simulink subsystem "complete_magnetic_model"  (R2023b)
settings: Solver=VariableStepAuto  StartTime=0.0  StopTime=10.0  RelTol=1e-3
undefined symbols (not defined in the file): astro_data, astroConstants, orbit_data, worldMag_data
settings Model: Creator=pierb  LastModifiedBy=pierb

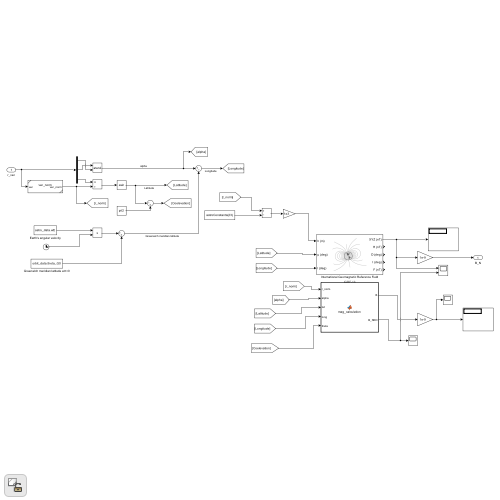
[thumbnail: Simulink's stored preview of the top-level diagram]
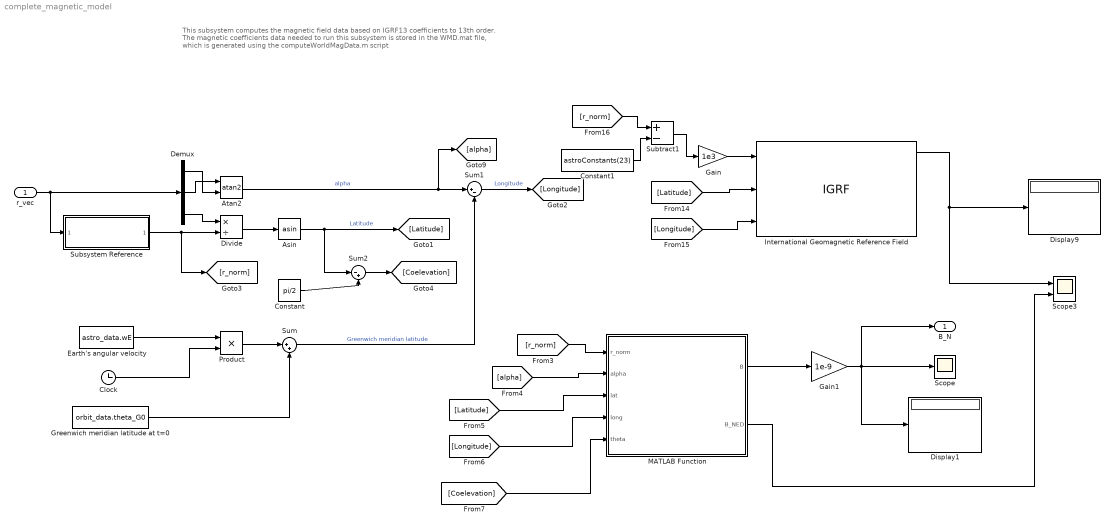
== system complete_magnetic_model ==
  note: This subsystem computes the magnetic
      | field data based on IGRF13 coefficients
      | to 13th order.
      | The magnetic coefficients data needed to run this subsystem is stored in the WMD.mat file, which is generated using the computeWorldMagData.m script
  r_vec : Inport
  Asin : Trigonometry  Operator=asin
  Atan2 : Trigonometry  Operator=atan2
  Clock : Clock
  Constant : Constant  Value=pi/2
  Constant1 : Constant  Value=astroConstants(23)
  Demux : Demux  Outputs=3
  Display1 : Display
  Display9 : Display
  Divide : Product  Inputs=*/
  Earth's angular velocity : Constant  Value=astro_data.wE
  Gain : Gain  Gain=1e3
  Gain1 : Gain  Gain=1e-9
  Greenwich meridian latitude at t=0 : Constant  Value=orbit_data.theta_G0
  International Geomagnetic Reference Field : IGRF  time_in=off  month=January  day=1  year=2020  sv_out=off
      settings: AttributesFormatString=%<generation>
  MATLAB Function : MATLAB Function  TreatAsAtomicUnit=on
  Product : Product
  Scope : Scope
  Scope3 : Scope  NumInputPorts=2
  Subsystem Reference : Subsystem  ReferencedSubsystem=vec_norm
  Subtract1 : Sum  Inputs=+-
  Sum : Sum  Inputs=|++
  Sum1 : Sum  Inputs=|+-
  Sum2 : Sum  Inputs=|-+
  B_N : Outport
  wires:
  Earth's angular velocity/1 -> Product/1
  Clock/1 -> Product/2
  Product/1 -> Sum/1
  Greenwich meridian latitude at t=0/1 -> Sum/2
  Sum/1 -> Sum1/2  "Greenwich meridian latitude"
  Demux/1 -> Atan2/2
  Demux/2 -> Atan2/1
  r_vec/1 -> Subsystem Reference/1, Demux/1
  Atan2/1 -> [alpha], Sum1/1  "alpha"
  Sum1/1 -> [Longitude]  "Longitude"
  Divide/1 -> Asin/1
  Demux/3 -> Divide/1
  Subsystem Reference/1 -> Divide/2, [r_norm]
  Asin/1 -> Sum2/1, [Latitude]  "Latitude"
  Constant/1 -> Sum2/2
  Sum2/1 -> [Coelevation]
  [r_norm] -> MATLAB Function/1(r_norm)
  [alpha] -> MATLAB Function/2(alpha)
  [Latitude] -> MATLAB Function/3(lat)
  [Longitude] -> MATLAB Function/4(long)
  [Coelevation] -> MATLAB Function/5(theta)
  MATLAB Function/1(B) -> Gain1/1
  MATLAB Function/2(B_NED) -> Scope3/2
  [Latitude] -> International Geomagnetic Reference Field/2
  [Longitude] -> International Geomagnetic Reference Field/3
  [r_norm] -> Subtract1/1
  Constant1/1 -> Subtract1/2
  Subtract1/1 -> Gain/1
  Gain/1 -> International Geomagnetic Reference Field/1
  International Geomagnetic Reference Field/1 -> Display9/1, Scope3/1
  Gain1/1 -> B_N/1, Scope/1, Display1/1

== matlab function complete_magnetic_model/MATLAB Function ==
  data: B output; r_norm input; alpha input; lat input; long input; theta input; B_NED output; worldMag_data parameter; astro_data parameter
function [B, B_NED] = mag_calculation(r_norm, alpha, lat, long, theta, worldMag_data, astro_data)

N = worldMag_data.N;
K = worldMag_data.K;
g = worldMag_data.g;
h = worldMag_data.h;
R = astroConstants(23);
el = astro_data.eps;

%% P Calculation
P = zeros(N, N+1);
% P_00
P_00 = 1;
P(1,1) = cos(theta) * P_00; % P_1,0: n=1, m=0
P(1,2) = sin(theta) * P_00; % P_1,1: n=1, m=1

for n = 2:N
    for m = 0:n
        if n == 2 && m ~= n
            P(n, m+1) = cos(theta)*P(n-1, m+1) - K(n, m+1) * P_00;
        else
            if m == n
                P(n, m+1) = sin(theta)*P(n-1, m);
            else
                P(n, m+1) = cos(theta)*P(n-1, m+1) - K(n, m+1) * P(n-2, m+1);
            end
        end
    end
end

%% dP/dTh calculation

dP = zeros(N, N+1);
dP_00 = 0;

dP(1,1) = -sin(theta)*P_00; % dP_1,0: n=1, m=0
dP(1,2) = cos(theta)*P_00;  % dP_1,1: n=1, m=1

for n = 2:N
    for m = 0:n
        if n == 2 && m ~= n
            dP(n, m+1) = cos(theta)*dP(n-1, m+1) - sin(theta)*P(n-1, m+1);
        else
            if m==n
                dP(n, m+1) = sin(theta)*dP(n-1, m) + cos(theta)*P(n-1,m);
            else
                dP(n, m+1) = cos(theta)*dP(n-1, m+1) - sin(theta)*P(n-1, m+1) - K(n, m+1)*dP(n-2, m+1);
            end
        end
    end
end

%% Magnetic field

Br = 0;
Bth = 0;
Bph = 0;

for n = 1:N
    Br_n = (R/r_norm)^(n+2)*(n+1); 
    Br_m = 0;

    Bth_n = (R/r_norm)^(n+2);
    Bth_m = 0;

    Bph_n = (R/r_norm)^(n+2);
    Bph_m = 0;
    for m = 0:N
        Br_m = Br_m + (g(n, m+1)*cos(m*long) + h(n, m+1)*sin(m*long))*P(n, m+1);
        Bth_m = Bth_m + (g(n, m+1)*cos(m*long) + h(n, m+1)*sin(m*long))*dP(n, m+1);
        Bph_m = Bph_m + (-m*g(n, m+1)*sin(m*long) + m*h(n, m+1)*cos(m*long))*P(n, m+1);
    end
    Br = Br + Br_n*Br_m;
    Bth = Bth + Bth_n*Bth_m;
    Bph = Bph + Bph_n*Bph_m;
end

Bth = -Bth;
Bph = -1/sin(theta)*Bph;

%% change frame

B_x = (Br*cos(lat) + Bth*sin(lat))*cos(alpha) - Bph*sin(alpha);
B_y = (Br*cos(lat) + Bth*sin(lat))*sin(alpha) + Bph*cos(alpha);
B_z = Br*sin(lat) - Bth*cos(lat);

B = [B_x; B_y; B_z];

%% NED

B_N = -Bth*cos(el) - Br*sin(el);
B_E = Bph;
B_D = Bth*sin(el) - Br*cos(el);

B_NED = [B_N B_E B_D];

end
